simulink model "HL_control_pos_FFforce_RC_WirtualWall_Sync"  (R2020a)
settings: Solver=ode4  StartTime=0.0  StopTime=inf  FixedStep=0.001  RelTol=1e-3
libraries: xpcethercatlib x42, simulink x12, slrtlib x10, AssistOn_Gait_Lib x6
(part 3 of 3)

== stateflow chart HL_control_pos_FFforce_RC_WirtualWall_Sync/High-Level Controller/System Enable ==
  settings: sampleTime=0.001
  state MaintainCommunication [parallel]
    init_ethercat();
    settings: executionOrder=1
    state init_ethercat [function]
  state ErrorHandling [parallel]
    settings: executionOrder=2
    state Device [parallel]
      entry:   sysON = false;
      during:
      stat = check_status();
      % If any disk position exeeds the soft limit, the corresponding element of `stopREF` is set to the
      % soft limit value. Othervise, the disk is in safe region and the element is zero.
      stopREF = limit_exceeded(diskpos);
      % The reference position is generated for convenience. A position control algorithm can be employed
      % to push the exceeding disk into the operational space and
      settings: executionOrder=2
      state Fault
      state SwitchOnDisabled
      state Init
      state Ready2SwitchOn
      state LimitExceeded
      state OperationEnabled
        entry, during:
        sysON = true;
        exit:
        sysON = false;
      state s = check_status [function]
      Fault -> SwitchOnDisabled : [all(stat == 64)]
      SwitchOnDisabled -> Ready2SwitchOn [order 1] : [all(stat == 33)]
      (junction 72) -> SwitchOnDisabled [order 2] : [all(stat == 64)]
      SwitchOnDisabled -> (junction 72) [order 2]
      (junction 85) -> Fault [order 1] : [any(stat == 8)]
      (default) -> Init
      Init -> (junction 85)
      (junction 85) -> (junction 72) [order 2]
      (junction 72) -> Ready2SwitchOn [order 3] : [all(stat == 33)]
      LimitExceeded -> (junction 85) : after(1, sec)
      OperationEnabled -> (junction 85)
      (junction 72) -> LimitExceeded [order 1] : [any(stopREF)]
      Ready2SwitchOn -> OperationEnabled : [all(stat == 55)]
    state Action [parallel]
      settings: executionOrder=1
      state set_control_word(c) [function]
      state ClearError
        state SetBit8Low
          set_control_word(0);
        state ClearFault
          set_control_word(128);
        state Wait4StateChange
        SetBit8Low -> ClearFault
        ClearFault -> Wait4StateChange
      state Wait4LimitSafe
      state MakeReady
        entry:
        set_control_word(6);
      state Idle
      state SwitchOnEnable
        set_control_word(15);
      Action -> SetBit8Low : [hasChanged(clear)]
      Wait4StateChange -> MakeReady : [in(Device.SwitchOnDisabled)]
      Wait4LimitSafe -> Idle : [~in(Device.LimitExceeded)]
      (junction 107) -> Wait4LimitSafe [order 1] : [in(Device.LimitExceeded)]
      Idle -> (junction 107)
      (junction 107) -> MakeReady [order 3] : [in(Device.SwitchOnDisabled)]
      (default) -> Idle
      (junction 107) -> SwitchOnEnable [order 2] : after(2, sec)[in(Device.Ready2SwitchOn)]
      SwitchOnEnable -> Idle
      MakeReady -> SwitchOnEnable : [in(Device.Ready2SwitchOn)]
  data: s function_output double size=[6 1]; rrp function_input; ref function_output double size=[6 1]; c function_input double size=1; sysON output boolean size=1; diskpos input Bus: AllDiskPos size=1; stat output double size=[6 1]; clear input; stopREF local double size=[6 1]
  function ref = limit_exceeded(rrp):
    | function ref = limit_exceeded(rrp)
    | % Checks if any of the disk angles of the 3RRPs exceeded the soft limits
    | % defined below.
    | 
    | % Get the disk angles.
    | q = [rrp.right;
    |      rrp.left];
    | % Clear the initial conditions
    | q = q - [pi/3; pi; -pi/3; pi/3; pi; -pi/3];
    | 
    | % Set the limits in DEGREES! Initial position is assumed to be zero
    | stop = 150;
    | lo_lims = -stop .* ones(6, 1) * (pi/180);
    | hi_lims =  stop .* ones(6, 1) * (pi/180);
    | 
    | lb = q < lo_lims;
    | ref = lb .* lo_lims;
    | 
    | hb = q > hi_lims;
    | ref = ref + hb .* hi_lims;

== stateflow chart HL_control_pos_FFforce_RC_WirtualWall_Sync/High-Level Feedback/Heel Sensor ==
  settings: sampleTime=0.001
  state Heel
    entry:
    gait.period = 0;
    gait.heelstriked.right = 0;
    gait.heelstriked.left = 0;
    state b = contacted(side) [function]
      (junction 398) -> (junction 393) : {b = heel_force.right > contact_threshold}
      (junction 390) -> (junction 398) [order 1] : [side == 'R']
      (default) -> (junction 390)
      (junction 390) -> (junction 395) [order 2] : {b = heel_force.left > contact_threshold}
    state t = estimate_stride [function]
      note: Average of stride times of both legs. Both legs should perform a full stride to estimate the average. If one of the legs does not complete a full strike, then its stride time is zero. Then use only one of the stride times.
      (default) -> (junction 464) : {t = (t_stride_r + t_stride_l) / (1 + full_stride_r * full_stride_l);}
    state Right [parallel]
      settings: executionOrder=1
      state Init
        t_ground_r = 0;
        t_off_r = 0;
        t_stride_r = 0;
        t_stride_p_r = t_stride_max;
        ground_1st_contact_r = 0;
        ground_1st_off_r = 0;
        full_stride_r = 0;
      state GroundContact
        gait.heelstriked.right = 0;
        ground_1st_contact_r = 1;
        t_ground_r = elapsed(sec);
      state Off
        ground_1st_off_r = 1;
        t_off_r = elapsed(sec);
      state Strike
        full_stride_r = ground_1st_contact_r * ground_1st_off_r;
        t_stride_c_r = (t_ground_r + t_off_r) * full_stride_r;
        t_stride_r = full_stride_r * (0.7*t_stride_c_r + 0.3*t_stride_p_r);
        t_stride_p_r = t_stride_c_r;
        gait.period = estimate_stride();
        gait.heelstriked.right = full_stride_r;
      (default) -> Heel.Right.Init
      Heel.Right.Off -> Heel.Right.Init [order 2] : [t_off_r > t_stride_max / 2]
      Heel.Right.Init -> (junction 113)
      (junction 113) -> Heel.Right.GroundContact [order 1] : [contacted('R')]
      (junction 113) -> Heel.Right.Off [order 2]
      Heel.Right.GroundContact -> Heel.Right.Init [order 2] : [t_ground_r > t_stride_max / 2]
      Heel.Right.GroundContact -> Heel.Right.Off [order 1] : [~contacted('R')]
      Heel.Right.Off -> Heel.Right.Strike [order 1] : [contacted('R')]
      Heel.Right.Strike -> Heel.Right.GroundContact
    state Left [parallel]
      settings: executionOrder=2
      state Init
        t_ground_l = 0;
        t_off_l = 0;
        t_stride_l = 0;
        t_stride_p_l = t_stride_max;
        ground_1st_contact_l = 0;
        ground_1st_off_l = 0;
        full_stride_l = 0;
      state GroundContact
        gait.heelstriked.left = 0;
        ground_1st_contact_l = 1;
        t_ground_l = elapsed(sec);
      state Off
        ground_1st_off_l = 1;
        t_off_l = elapsed(sec);
      state Strike
        full_stride_l = ground_1st_contact_l * ground_1st_off_l;
        t_stride_c_l = (t_ground_l + t_off_l) * full_stride_l;
        t_stride_l = full_stride_l * (0.7*t_stride_c_l + 0.3*t_stride_p_l);
        t_stride_p_l = t_stride_c_l;
        gait.period = estimate_stride();
        gait.heelstriked.left = full_stride_l;
      (default) -> Heel.Left.Init
      Heel.Left.Off -> Heel.Left.Init [order 2] : [t_off_l > t_stride_max / 2]
      Heel.Left.Init -> (junction 174)
      (junction 174) -> Heel.Left.GroundContact [order 1] : [contacted('L')]
      (junction 174) -> Heel.Left.Off [order 2]
      Heel.Left.GroundContact -> Heel.Left.Init [order 2] : [t_ground_l > t_stride_max / 2]
      Heel.Left.GroundContact -> Heel.Left.Off [order 1] : [~contacted('L')]
      Heel.Left.Off -> Heel.Left.Strike [order 1] : [contacted('L')]
      Heel.Left.Strike -> Heel.Left.GroundContact
  data: side function_input; b function_output; t function_output; heel_force input Bus: HeelForce size=1; contact_threshold constant double =2.5; t_stride_max constant double =3; ground_1st_contact_r local double size=1; t_ground_r local double size=1; t_off_r local double size=1; t_stride_p_r local double size=1; ground_1st_contact_l local double size=1; ground_1st_off_l local double size=1; t_ground_l local double size=1; t_off_l local double size=1; t_stride_p_l local double size=1; full_stride_r local double size=1; ground_1st_off_r local double size=1; t_stride_c_r local double size=1; full_stride_l local double size=1; t_stride_c_l local double size=1; t_stride_l local double size=1; t_stride_r local double size=1; gait output Bus: Gait size=1

== matlab function HL_control_pos_FFforce_RC_WirtualWall_Sync/Vırtual Wall Referance/MATLAB Function ==
  data: pos input; pos output; vel input; vel output
function [pos, vel] = rotate2HMIcoordsPOS(pos, vel)
r = 0.254574 + pi;
RzT = [cos(r) -sin(r) 0;
       sin(r)  cos(r) 0;
        0        0    1]';

xy = RzT * [pos(1:2) vel(1:2); 1 1];

pos(1:2) = xy(1:2, 1);
vel(1:2) = xy(1:2, 2);

== matlab function HL_control_pos_FFforce_RC_WirtualWall_Sync/Right Leg/Velocity Sourced Compansator/MATLAB Function1 ==
  data: Vel input; Torque output; MaxGain input; Mode input
function Torque = NegativeDampingController(Vel,MaxGain,Mode)

Disk1 = Vel(1);
Disk2 = Vel(2);
Disk3 = Vel(3);

beta =  MaxGain(1);
alpha = MaxGain(2);
gamma = MaxGain(3);

if Disk1 < -0.05 || Disk1 > 0.05
   Coef1 = 0;
else 
Coef1 = -beta + abs(beta*tanh(Disk1));
end

if Disk2 < -0.05 || Disk2 > 0.05
   Coef2 = 0;
else 
Coef2 = -alpha + abs(alpha*tanh(Disk2));
end

if Disk3 < -0.05 || Disk3 > 0.05
   Coef3 = 0;
else 
Coef3 = -gamma + abs(gamma*tanh(Disk3));
end

Torque = zeros(3,1);

if Mode == 2 
Torque(1) = -Coef1 * Disk1;
Torque(2) = -Coef2 * Disk2;
Torque(3) = -Coef3 * Disk3;
end

== matlab function HL_control_pos_FFforce_RC_WirtualWall_Sync/Left Leg/Velocity Sourced Compansator/MATLAB Function1 ==
  data: Vel input; Torque output; MaxGain input; Mode input
function Torque = NegativeDampingController(Vel,MaxGain,Mode)

Disk1 = Vel(1);
Disk2 = Vel(2);
Disk3 = Vel(3);

beta =  MaxGain(1);
alpha = MaxGain(2);
gamma = MaxGain(3);

if abs(Disk1) > 0.05
   Coef1 = 0;
else 
Coef1 = -beta + abs(beta*tanh(Disk1));
end

if abs(Disk2) > 0.05
   Coef2 = 0;
else 
Coef2 = -alpha + abs(alpha*tanh(Disk2));
end

if abs(Disk3) > 0.05
   Coef3 = 0;
else 
Coef3 = -gamma + abs(gamma*tanh(Disk3));
end

Torque = zeros(3,1);

if Mode == 2 
Torque(1) = -Coef1 * Disk1;
Torque(2) = -Coef2 * Disk2;
Torque(3) = -Coef3 * Disk3;
end
